simulink model "New_try_angular"  (R2020b)
settings: Solver=VariableStepAuto  StartTime=0.0  StopTime=3  RelTol=1e-3
undefined symbols (not defined in the file): I_inv, I_mat, I_xx, I_xz, I_yy, I_zz
libraries: vrlib x2
settings Model: Creator=Jonathan van Zyl  LastModifiedBy=Jonathan van Zyl

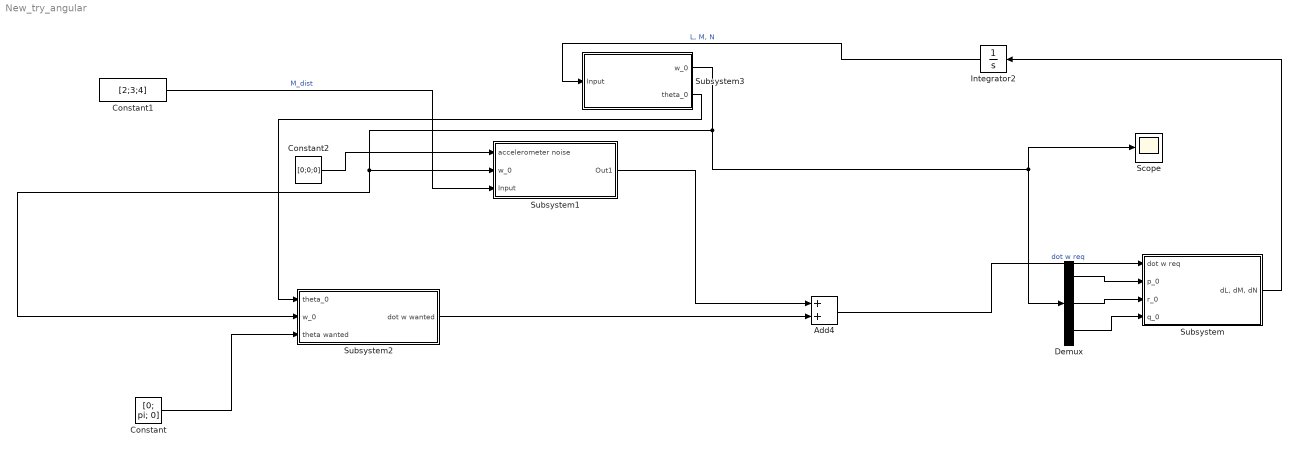
== system New_try_angular ==
  Add4 : Sum
  Constant : Constant  Value=[0; pi; 0]
  Constant1 : Constant  Value=[2;3;4]
  Constant2 : Constant  Value=[0;0;0]
  Demux : Demux  Outputs=3
  Integrator2 : Integrator  InitialCondition=[0;0;0]
  Scope : Scope
  Subsystem : Subsystem
  Subsystem1 : Subsystem
  Subsystem2 : Subsystem
  Subsystem3 : Subsystem
  wires:
  Add4/1 -> Subsystem/1(dot w req)  "dot w req"
  Subsystem/1("dL, dM, dN") -> Integrator2/1
  Subsystem1/1(Out1) -> Add4/1
  Subsystem2/1(dot w wanted) -> Add4/2
  Constant/1 -> Subsystem2/3(theta wanted)
  Constant2/1 -> Subsystem1/1(accelerometer noise)
  Integrator2/1 -> Subsystem3/1(Input)  "L, M, N"
  Subsystem3/1(w_0) -> Demux/1, Scope/1, Subsystem2/2(w_0), Subsystem1/2(w_0)
  Subsystem3/2(theta_0) -> Subsystem2/1(theta_0)
  Demux/1 -> Subsystem/2(p_0)
  Demux/2 -> Subsystem/3(r_0)
  Demux/3 -> Subsystem/4(q_0)
  Constant1/1 -> Subsystem1/3(Input)  "M_dist"

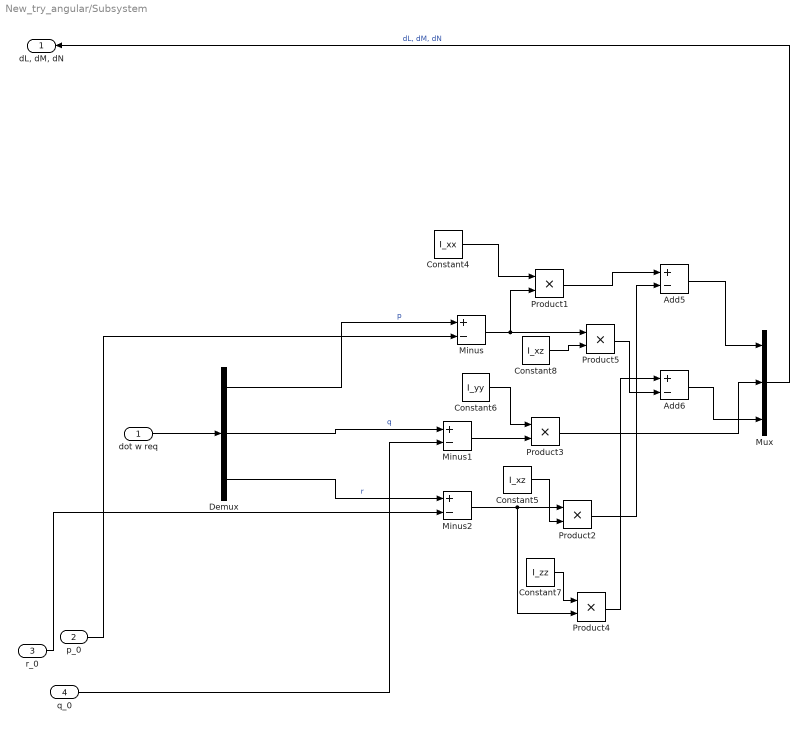
== system New_try_angular/Subsystem ==
  dot w req : Inport
  p_0 : Inport  Port=2
  r_0 : Inport  Port=3
  q_0 : Inport  Port=4
  Add5 : Sum  Inputs=+-
  Add6 : Sum  Inputs=+-
  Constant4 : Constant  Value=I_xx
  Constant5 : Constant  Value=I_xz
  Constant6 : Constant  Value=I_yy
  Constant7 : Constant  Value=I_zz
  Constant8 : Constant  Value=I_xz
  Demux : Demux  Outputs=3
  Minus : Sum  Inputs=+-
  Minus1 : Sum  Inputs=+-
  Minus2 : Sum  Inputs=+-
  Mux : Mux  Inputs=3
  Product{1..5} (5 alike) : Product
  "dL, dM, dN" : Outport
  wires:
  Constant8/1 -> Product5/2
  Product5/1 -> Add6/2
  Add5/1 -> Mux/1
  dot w req/1 -> Demux/1
  Minus2/1 -> Product4/2, Product2/1
  Product1/1 -> Add5/1
  Constant4/1 -> Product1/1
  Demux/1 -> Minus/1  "p"
  Minus1/1 -> Product3/2
  Product3/1 -> Mux/2
  Product4/1 -> Add6/1
  Minus/1 -> Product1/2, Product5/1
  Demux/2 -> Minus1/1  "q"
  q_0/1 -> Minus1/2
  Product2/1 -> Add5/2
  Constant6/1 -> Product3/1
  Add6/1 -> Mux/3
  Demux/3 -> Minus2/1  "r"
  Constant5/1 -> Product2/2
  p_0/1 -> Minus/2
  Constant7/1 -> Product4/1
  Mux/1 -> "dL, dM, dN"/1  "dL, dM, dN"
  r_0/1 -> Minus2/2

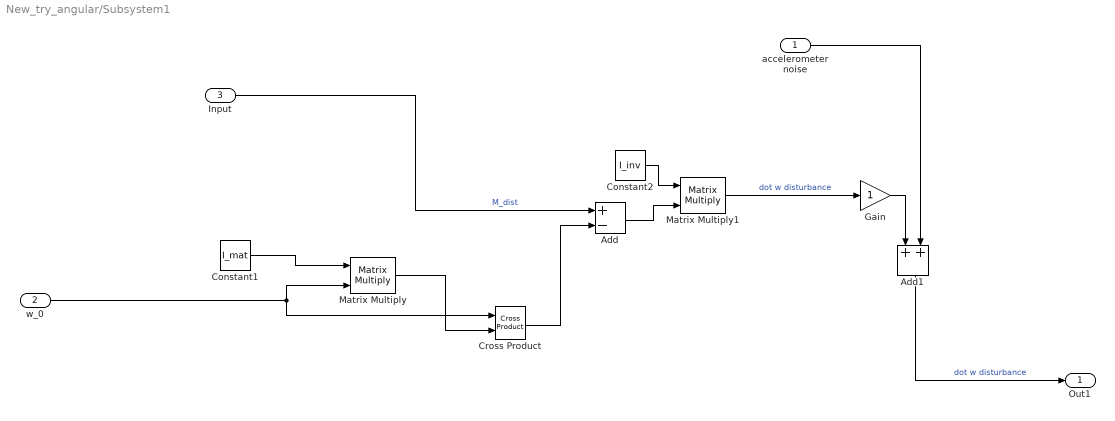
== system New_try_angular/Subsystem1 ==
  accelerometer noise : Inport
  w_0 : Inport  Port=2
  Input : Inport  Port=3
  Add : Sum  Inputs=+-
  Add1 : Sum
  Constant1 : Constant  Value=I_mat
  Constant2 : Constant  Value=I_inv
  Cross Product : vrlib/Utilities/Cross Product
  Gain : Gain
  Matrix Multiply : Product  Multiplication=Matrix(*)
  Matrix Multiply1 : Product  Multiplication=Matrix(*)
  Out1 : Outport
  wires:
  Add1/1 -> Out1/1  "dot w disturbance"
  Gain/1 -> Add1/1
  Matrix Multiply/1 -> Cross Product/2
  Add/1 -> Matrix Multiply1/2
  Matrix Multiply1/1 -> Gain/1  "dot w disturbance"
  w_0/1 -> Cross Product/1, Matrix Multiply/2
  Cross Product/1 -> Add/2
  Constant1/1 -> Matrix Multiply/1
  Constant2/1 -> Matrix Multiply1/1
  Input/1 -> Add/1  "M_dist"
  accelerometer noise/1 -> Add1/2

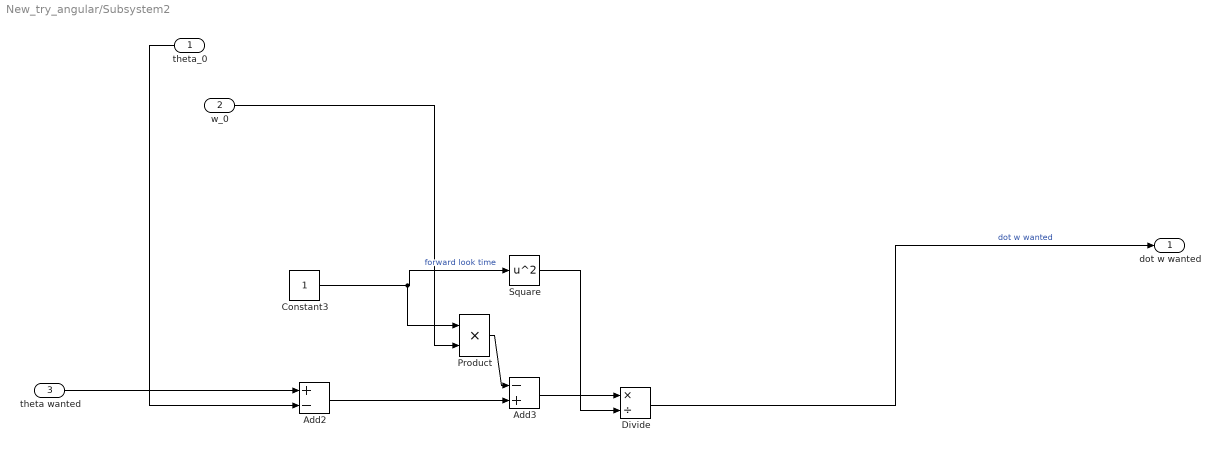
== system New_try_angular/Subsystem2 ==
  theta_0 : Inport
  w_0 : Inport  Port=2
  theta wanted : Inport  Port=3
  Add2 : Sum  Inputs=+-
  Add3 : Sum  Inputs=-+
  Constant3 : Constant
  Divide : Product  Inputs=*/
  Product : Product
  Square : Math  Operator=square  SaturateOnIntegerOverflow=on
  dot w wanted : Outport
  wires:
  Add2/1 -> Add3/2
  Divide/1 -> dot w wanted/1  "dot w wanted"
  Square/1 -> Divide/2
  Constant3/1 -> Square/1, Product/1  "forward look time"
  theta wanted/1 -> Add2/1
  Add3/1 -> Divide/1
  Product/1 -> Add3/1
  theta_0/1 -> Add2/2
  w_0/1 -> Product/2

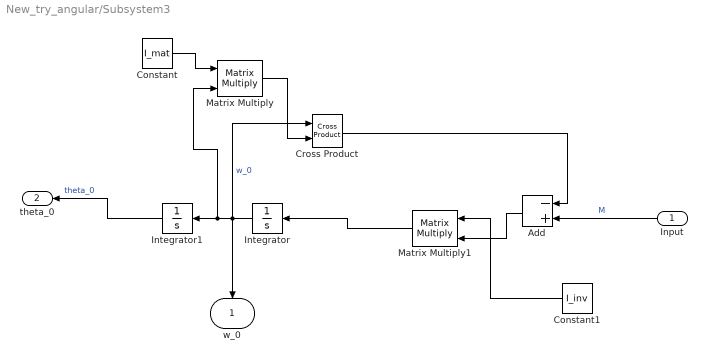
== system New_try_angular/Subsystem3 ==
  Input : Inport
  Add : Sum  Inputs=-+
  Constant : Constant  Value=I_mat
  Constant1 : Constant  Value=I_inv
  Cross Product : vrlib/Utilities/Cross Product
  Integrator : Integrator  InitialCondition=[0;0;0]
  Integrator1 : Integrator  InitialCondition=[0;0;0]
  Matrix Multiply : Product  Multiplication=Matrix(*)
  Matrix Multiply1 : Product  Multiplication=Matrix(*)
  w_0 : Outport
  theta_0 : Outport  Port=2
  wires:
  Integrator/1 -> Cross Product/1, w_0/1, Matrix Multiply/2, Integrator1/1  "w_0"
  Matrix Multiply1/1 -> Integrator/1
  Integrator1/1 -> theta_0/1  "theta_0"
  Input/1 -> Add/2  "M"
  Cross Product/1 -> Add/1
  Constant/1 -> Matrix Multiply/1
  Matrix Multiply/1 -> Cross Product/2
  Constant1/1 -> Matrix Multiply1/1
  Add/1 -> Matrix Multiply1/2
